simulink model "demo_filters_low_and_high_input_bandlimited_whitenoise"  (Simulink 7.8)
settings: Solver=ode45  StartTime=0.0  StopTime=10.0  RelTol=1e-3
libraries: simulink x1
settings Model: Creator=Ramanathan  LastModifiedBy=Ramanathan

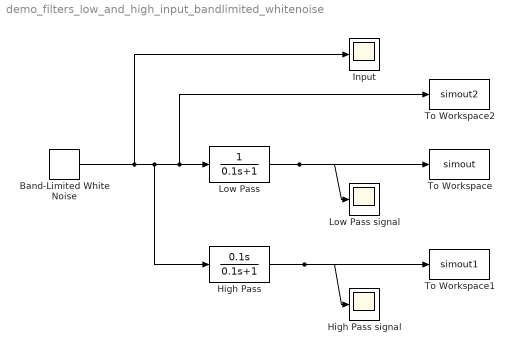
== system demo_filters_low_and_high_input_bandlimited_whitenoise ==
  Band-Limited White Noise : simulink/Sources/Band-Limited White Noise  Cov=[0.1]  Ts=0.1  seed=[23341]
  High Pass : TransferFcn  Numerator=[0.1 0]  Denominator=[0.1 1]
  High Pass signal : Scope
      settings: SaveName=ScopeData2
  Input : Scope
  Low Pass : TransferFcn  Denominator=[0.1 1]
  Low Pass signal : Scope
  To Workspace : ToWorkspace  VariableName=simout  SampleTime=-1  SaveFormat=Structure
  To Workspace1 : ToWorkspace  VariableName=simout1  SampleTime=-1  SaveFormat=Structure
  To Workspace2 : ToWorkspace  VariableName=simout2  SampleTime=-1  SaveFormat=Structure
  wires:
  Band-Limited White Noise/1 -> Input/1, High Pass/1, Low Pass/1, To Workspace2/1
  Low Pass/1 -> Low Pass signal/1, To Workspace/1
  High Pass/1 -> High Pass signal/1, To Workspace1/1
